simulink model "Pitch_Angular"  (R2016b)
settings: Solver=VariableStepAuto  StartTime=0.0  StopTime=10.0  RelTol=1e-3
settings Model: Creator=Administrator  LastModifiedBy=Administrator

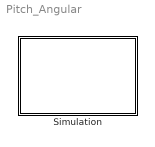
== system Pitch_Angular ==
  Simulation : Subsystem  mask{kp=4.00, ki=10.8, k1=0.4103, k2=3.1623}

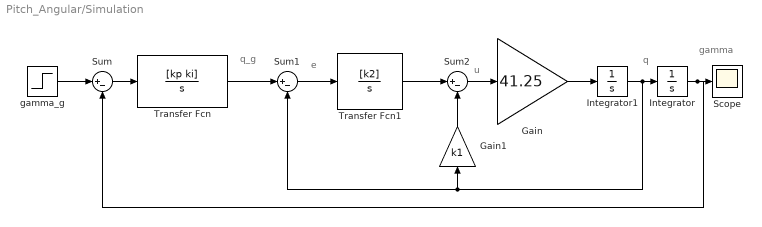
== system Pitch_Angular/Simulation ==
  note: q
  note: u
  note: e
  note: q_g
  note: gamma
  Gain : Gain  Gain=41.25
  Gain1 : Gain  Gain=k1
  Integrator : Integrator
  Integrator1 : Integrator
  Scope : Scope
  Sum : Sum  Inputs=|+-
  Sum1 : Sum  Inputs=|+-
  Sum2 : Sum  Inputs=|+-
  Transfer Fcn : TransferFcn  Numerator=[kp ki]  Denominator=[1 0]
  Transfer Fcn1 : TransferFcn  Numerator=[k2]  Denominator=[1 0]
  gamma_g : Step  Time=0  SampleTime=0
  wires:
  Integrator1/1 -> Sum1/2, Gain1/1, Integrator/1
  Transfer Fcn1/1 -> Sum2/1
  Transfer Fcn/1 -> Sum1/1
  gamma_g/1 -> Sum/1
  Sum2/1 -> Gain/1
  Integrator/1 -> Sum/2, Scope/1
  Gain/1 -> Integrator1/1
  Gain1/1 -> Sum2/2
  Sum1/1 -> Transfer Fcn1/1
  Sum/1 -> Transfer Fcn/1
